simulink model "Book331"  (R2019b)
settings: Solver=FixedStepAuto  StartTime=0  StopTime=100  FixedStep=0.001  RelTol=1e-3  EnableMultiTasking=on
settings Model: Creator=xyh  LastModifiedBy=user
settings DataIOCC: ReturnWorkspaceOutputs=off
settings OptimizationCC: LifeSpan=inf
settings DebuggingCC: SFUnexpectedBacktrackingDiag=warning  SFNoUnconditionalDefaultTransitionDiag=warning  ArithmeticOperatorsInVariantConditions=warning
settings SFSimCC: SimUseLocalCustomCode=off  CustomCodeUndefinedFunction=UseInterfaceOnly
settings RTWCC: RTWUseLocalCustomCode=off
settings CodeAppCC: StateflowObjectComments=on
settings GRTTargetCC: TargetLangStandard=C89/C90 (ANSI)  GeneratePreprocessorConditionals=Disable all
settings ConfigComp: CovMetricSettings=dw  CovHtmlReporting=on  CovSaveCumulativeToWorkspaceVar=on  CovSaveSingleToWorkspaceVar=on  CovExternalEMLEnable=off

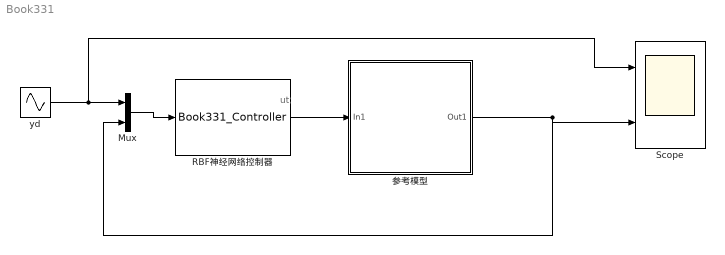
== system Book331 ==
  note: ut
  Mux : Mux  Inputs=2
  RBF神经网络控制器 : S-Function  FunctionName=Book331_Controller  SFunctionDeploymentMode=off  EnableBusSupport=off
  Scope : Scope  NumInputPorts=2
  yd : Sin  Amplitude=2  Frequency=0.1*pi  SampleTime=0
  参考模型 : Subsystem
  wires:
  yd/1 -> Scope/1, Mux/1
  RBF神经网络控制器/1 -> 参考模型/1(In1)
  参考模型/1(Out1) -> Scope/2, Mux/2
  Mux/1 -> RBF神经网络控制器/1

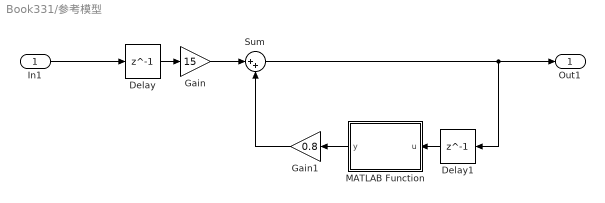
== system Book331/参考模型 ==
  In1 : Inport
  Delay : Delay  DelayLength=1  InitialCondition=0
  Delay1 : Delay  DelayLength=1  InitialCondition=0
  Gain : Gain  Gain=15
  Gain1 : Gain  Gain=0.8
  MATLAB Function : MATLAB Function  TreatAsAtomicUnit=on
  Sum : Sum  Inputs=|++
  Out1 : Outport
  wires:
  In1/1 -> Delay/1
  Sum/1 -> Delay1/1, Out1/1
  Gain/1 -> Sum/1
  Delay/1 -> Gain/1
  Delay1/1 -> MATLAB Function/1(u)
  Gain1/1 -> Sum/2
  MATLAB Function/1(y) -> Gain1/1

== matlab function Book331/参考模型/MATLAB Function ==
  data: u input; y output
function y = fcn(u)
%#codegen

y = sin(u);
